simulink library "full_bridge_three_level_ttype_mosfet_based_model"  (R2026a)
settings: Solver=VariableStepAuto
undefined symbols (not defined in the file): tc
libraries: fl_lib x88, nesl_utility x56, ee_lib x8
(part 1 of 2)
settings Model: Creator=dbagn  LastModifiedBy=d.bagnara

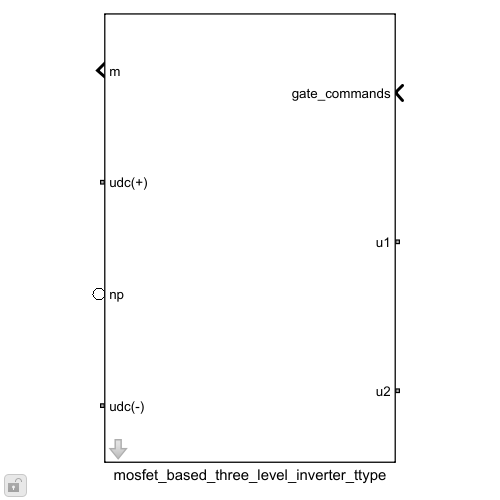
[thumbnail: Simulink's stored preview of the top-level diagram]
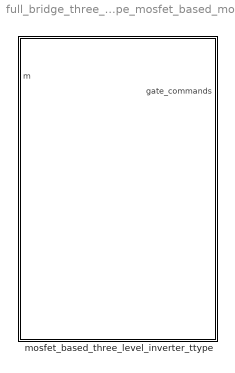
== system full_bridge_three_level_ttype_mosfet_based_model ==
  mosfet_based_three_level_inverter_ttype : Subsystem  mask{Vth_m=5.5, Rds_on_m=0.15e-3, Eon_m=200e-3, Eoff_m=300e-3, Erec_m=200e-3, Ion_sw_loss_m=900, Voff_sw_loss_m=900, Vdon_diode_m=2, Rdon_diode_m=0.15e-3, rth_mosfet_JH_m=0.018, rth_mosfet_HA_m=0.034, Csnubber_m=10e-9, Rsnubber_m=2200, JunctionTermalMass_m=2, mass_heatsink_m=0.15, specific_heat_m=880, Tambient_m=40, DThs_init_m=0, tc_m=tc}
      mask prompts: Vth_m "Vth (V)"; Rds_on_m "Rds_on (Ohm)"; Eon_m "Eon (J)"; Eoff_m "Eoff (J)"; Erec_m "Erec (J)"; Ion_sw_loss_m "Ion_sw_loss (A)"; Voff_sw_loss_m "Voff_sw_loss (V)"; Vdon_diode_m "Vdon_diode (V)"; Rdon_diode_m "Rdon_diode (Ohm)"; rth_mosfet_JH_m "rth_mosfet_JH (K/W)"; rth_mosfet_HA_m "rth_mosfet_HA  (K/W)"; Csnubber_m "Csnubber (F)"; Rsnubber_m "Rsnubber (Ohm)"; JunctionTermalMass_m "JunctionTermalMass (J/K)"; mass_heatsink_m "mass_heatsink (Kg)"; specific_heat_m "specific_heat (J/(K*Kg))"; Tambient_m "Tambient (Celsius)"; DThs_init_m "DThs_init (Celsius)"; tc_m "tc (s)"
      mask DialogControl inv Prompt: MOSFET
      mask DialogControl thermal Prompt: Thermal
      mask DialogControl sampling_time Prompt: Sampling time (s)

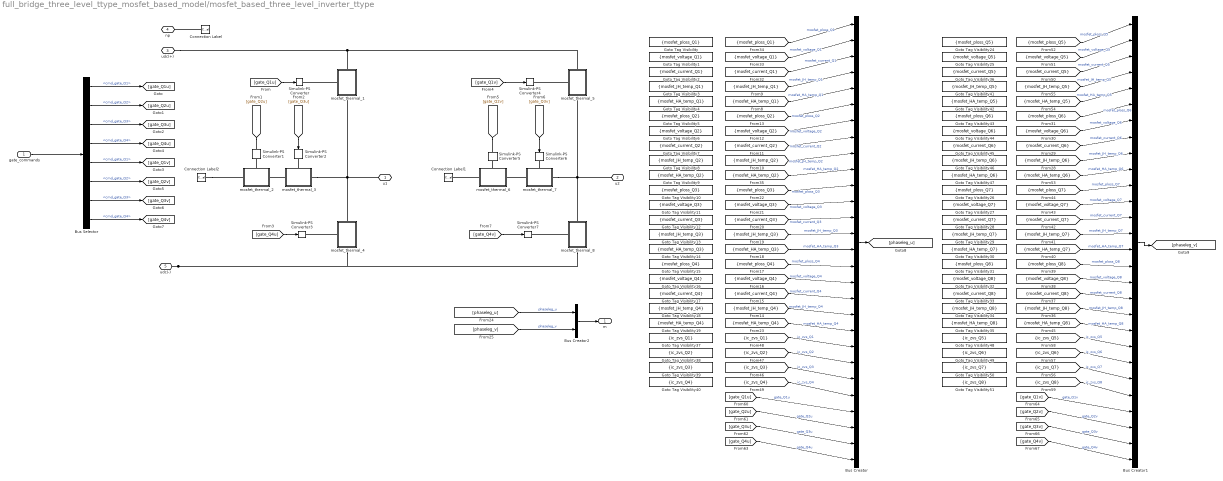
== system full_bridge_three_level_ttype_mosfet_based_model/mosfet_based_three_level_inverter_ttype ==
  gate_commands : Inport
  Bus Creator : BusCreator  Inputs=28
  Bus Creator1 : BusCreator  Inputs=28
  Bus Creator2 : BusCreator  Inputs=2
  Bus Selector : BusSelector  OutputSignals=gate_cmds_ph1.cmd_gate_Q1,gate_cmds_ph1.cmd_gate_Q2,gate_cmds_ph1.cmd_gate_Q3,gate_cmds_ph1.cmd_gate_Q4,gate_cmds_ph2.cmd_gate_Q1,gate_cmds_ph2.cmd_gate_Q2,gate_cmds_ph2.cmd_gate_Q3,gate_cmds_ph2.cmd_gate_Q4
  Connection Label : ConnectionLabel  Label=np
  Connection Label1 : ConnectionLabel  Label=np
  Connection Label2 : ConnectionLabel  Label=np
  Goto Tag Visibility : GotoTagVisibility  GotoTag=mosfet_ploss_Q1
  Goto Tag Visibility1 : GotoTagVisibility  GotoTag=mosfet_voltage_Q1
  Goto Tag Visibility10 : GotoTagVisibility  GotoTag=mosfet_ploss_Q3
  Goto Tag Visibility11 : GotoTagVisibility  GotoTag=mosfet_voltage_Q3
  Goto Tag Visibility12 : GotoTagVisibility  GotoTag=mosfet_current_Q3
  Goto Tag Visibility13 : GotoTagVisibility  GotoTag=mosfet_JH_temp_Q3
  Goto Tag Visibility14 : GotoTagVisibility  GotoTag=mosfet_HA_temp_Q3
  Goto Tag Visibility15 : GotoTagVisibility  GotoTag=mosfet_ploss_Q4
  Goto Tag Visibility16 : GotoTagVisibility  GotoTag=mosfet_voltage_Q4
  Goto Tag Visibility17 : GotoTagVisibility  GotoTag=mosfet_current_Q4
  Goto Tag Visibility18 : GotoTagVisibility  GotoTag=mosfet_JH_temp_Q4
  Goto Tag Visibility19 : GotoTagVisibility  GotoTag=mosfet_HA_temp_Q4
  Goto Tag Visibility2 : GotoTagVisibility  GotoTag=mosfet_current_Q1
  Goto Tag Visibility24 : GotoTagVisibility  GotoTag=mosfet_ploss_Q5
  Goto Tag Visibility25 : GotoTagVisibility  GotoTag=mosfet_voltage_Q5
  Goto Tag Visibility26 : GotoTagVisibility  GotoTag=mosfet_ploss_Q7
  Goto Tag Visibility27 : GotoTagVisibility  GotoTag=mosfet_voltage_Q7
  Goto Tag Visibility28 : GotoTagVisibility  GotoTag=mosfet_current_Q7
  Goto Tag Visibility29 : GotoTagVisibility  GotoTag=mosfet_JH_temp_Q7
  Goto Tag Visibility3 : GotoTagVisibility  GotoTag=mosfet_JH_temp_Q1
  Goto Tag Visibility30 : GotoTagVisibility  GotoTag=mosfet_HA_temp_Q7
  Goto Tag Visibility31 : GotoTagVisibility  GotoTag=mosfet_ploss_Q8
  Goto Tag Visibility32 : GotoTagVisibility  GotoTag=mosfet_voltage_Q8
  Goto Tag Visibility33 : GotoTagVisibility  GotoTag=mosfet_current_Q8
  Goto Tag Visibility34 : GotoTagVisibility  GotoTag=mosfet_JH_temp_Q8
  Goto Tag Visibility35 : GotoTagVisibility  GotoTag=mosfet_HA_temp_Q8
  Goto Tag Visibility36 : GotoTagVisibility  GotoTag=mosfet_current_Q5
  Goto Tag Visibility37 : GotoTagVisibility  GotoTag=ic_zvs_Q1
  Goto Tag Visibility38 : GotoTagVisibility  GotoTag=ic_zvs_Q2
  Goto Tag Visibility39 : GotoTagVisibility  GotoTag=ic_zvs_Q3
  Goto Tag Visibility4 : GotoTagVisibility  GotoTag=mosfet_HA_temp_Q1
  Goto Tag Visibility40 : GotoTagVisibility  GotoTag=ic_zvs_Q4
  Goto Tag Visibility41 : GotoTagVisibility  GotoTag=mosfet_JH_temp_Q5
  Goto Tag Visibility42 : GotoTagVisibility  GotoTag=mosfet_HA_temp_Q5
  Goto Tag Visibility43 : GotoTagVisibility  GotoTag=mosfet_ploss_Q6
  Goto Tag Visibility44 : GotoTagVisibility  GotoTag=mosfet_voltage_Q6
  Goto Tag Visibility45 : GotoTagVisibility  GotoTag=mosfet_current_Q6
  Goto Tag Visibility46 : GotoTagVisibility  GotoTag=mosfet_JH_temp_Q6
  Goto Tag Visibility47 : GotoTagVisibility  GotoTag=mosfet_HA_temp_Q6
  Goto Tag Visibility48 : GotoTagVisibility  GotoTag=ic_zvs_Q5
  Goto Tag Visibility49 : GotoTagVisibility  GotoTag=ic_zvs_Q6
  Goto Tag Visibility5 : GotoTagVisibility  GotoTag=mosfet_ploss_Q2
  Goto Tag Visibility50 : GotoTagVisibility  GotoTag=ic_zvs_Q7
  Goto Tag Visibility51 : GotoTagVisibility  GotoTag=ic_zvs_Q8
  Goto Tag Visibility6 : GotoTagVisibility  GotoTag=mosfet_voltage_Q2
  Goto Tag Visibility7 : GotoTagVisibility  GotoTag=mosfet_current_Q2
  Goto Tag Visibility8 : GotoTagVisibility  GotoTag=mosfet_JH_temp_Q2
  Goto Tag Visibility9 : GotoTagVisibility  GotoTag=mosfet_HA_temp_Q2
  Simulink-PS Converter{,1..7} (8 alike) : nesl_utility/Simulink-PS Converter  PhysicalDomain=network_engine_domain  SubClassName=ps_input  LeftPortType=input  RightPortType=output  PseudoPeriodic=off  Frequencies=[]  NoiseDistribution=none  NoiseParameters=[]  Unit=1  AffineConversion=on  FilteringAndDerivatives=provide  SimscapeFilterOrder=1  InputFilterTimeConstant=0.001  UdotUserProvided=0
  mosfet_thermal_1 : Subsystem
      settings: PortSchema="{\"entries\":[{\"content\":{\"sides\":[{\"content\":{\"connectorIds\":[\"LConn1\"]},\"type\":\"ConnectorPlacement.EquallySpacedRectSide\",\"uuid\":\"9277da8d-d460-43e6-8478-dd662f15d226\"},{\"content\":{\"connectorIds\":[],\"side\":\"RIGHT\"},\"type\":\"ConnectorPlacement.EquallySpacedRectSide\",\"uuid\":\"a7ece396-f1d9-4f4f-a05b-db1fc65d6e1d\"},{\"content\":{\"connectorIds\":[\"LConn2\"],\"side\":\"TOP\"},\"type\":\"ConnectorPlacement.EquallySpacedRectSide\",\"uuid\":\"fdd70777-e9cf-4317-afb6-cae87f75d5b0\"},{\"content\":{\"connectorIds\":[\"RConn1\"],\"side\":\"BOTTOM\"},\"type\":\"ConnectorPlacement.EquallySpacedRectSide\",\"uuid\":\"2353ed68-b1a1-4775-9ca9-31e268d5443b\"}]},\"type\":\"ConnectorPlacement.EquallySpacedConnector\",\"uuid\":\"d5479f4c-4e65-4791-adcb-73df11f88590\"}],\"packageUris\":[\"http://schema.mathworks.com/mf0/Connector/R2020b\"],\"version\":\"1.0\"}"
  mosfet_thermal_2 : Subsystem
      settings: PortSchema="{\"entries\":[{\"content\":{\"sides\":[{\"content\":{\"connectorIds\":[\"LConn1\"]},\"type\":\"ConnectorPlacement.EquallySpacedRectSide\",\"uuid\":\"9277da8d-d460-43e6-8478-dd662f15d226\"},{\"content\":{\"side\":\"RIGHT\"},\"type\":\"ConnectorPlacement.EquallySpacedRectSide\",\"uuid\":\"a7ece396-f1d9-4f4f-a05b-db1fc65d6e1d\"},{\"content\":{\"connectorIds\":[\"LConn2\"],\"side\":\"TOP\"},\"type\":\"ConnectorPlacement.EquallySpacedRectSide\",\"uuid\":\"fdd70777-e9cf-4317-afb6-cae87f75d5b0\"},{\"content\":{\"connectorIds\":[\"RConn1\"],\"side\":\"BOTTOM\"},\"type\":\"ConnectorPlacement.EquallySpacedRectSide\",\"uuid\":\"2353ed68-b1a1-4775-9ca9-31e268d5443b\"}]},\"type\":\"ConnectorPlacement.EquallySpacedConnector\",\"uuid\":\"d5479f4c-4e65-4791-adcb-73df11f88590\"}],\"packageUris\":[\"http://schema.mathworks.com/mf0/Connector/R2020b\"],\"version\":\"1.0\"}"
  mosfet_thermal_3 : Subsystem
      settings: PortSchema="{\"entries\":[{\"content\":{\"sides\":[{\"content\":{\"connectorIds\":[\"LConn1\"]},\"type\":\"ConnectorPlacement.EquallySpacedRectSide\",\"uuid\":\"9277da8d-d460-43e6-8478-dd662f15d226\"},{\"content\":{\"connectorIds\":[],\"side\":\"RIGHT\"},\"type\":\"ConnectorPlacement.EquallySpacedRectSide\",\"uuid\":\"a7ece396-f1d9-4f4f-a05b-db1fc65d6e1d\"},{\"content\":{\"connectorIds\":[\"LConn2\"],\"side\":\"TOP\"},\"type\":\"ConnectorPlacement.EquallySpacedRectSide\",\"uuid\":\"fdd70777-e9cf-4317-afb6-cae87f75d5b0\"},{\"content\":{\"connectorIds\":[\"RConn1\"],\"side\":\"BOTTOM\"},\"type\":\"ConnectorPlacement.EquallySpacedRectSide\",\"uuid\":\"2353ed68-b1a1-4775-9ca9-31e268d5443b\"}]},\"type\":\"ConnectorPlacement.EquallySpacedConnector\",\"uuid\":\"d5479f4c-4e65-4791-adcb-73df11f88590\"}],\"packageUris\":[\"http://schema.mathworks.com/mf0/Connector/R2020b\"],\"version\":\"1.0\"}"
  mosfet_thermal_4 : Subsystem
      settings: PortSchema="{\"entries\":[{\"content\":{\"sides\":[{\"content\":{\"connectorIds\":[\"LConn1\"]},\"type\":\"ConnectorPlacement.EquallySpacedRectSide\",\"uuid\":\"9277da8d-d460-43e6-8478-dd662f15d226\"},{\"content\":{\"connectorIds\":[],\"side\":\"RIGHT\"},\"type\":\"ConnectorPlacement.EquallySpacedRectSide\",\"uuid\":\"a7ece396-f1d9-4f4f-a05b-db1fc65d6e1d\"},{\"content\":{\"connectorIds\":[\"LConn2\"],\"side\":\"TOP\"},\"type\":\"ConnectorPlacement.EquallySpacedRectSide\",\"uuid\":\"fdd70777-e9cf-4317-afb6-cae87f75d5b0\"},{\"content\":{\"connectorIds\":[\"RConn1\"],\"side\":\"BOTTOM\"},\"type\":\"ConnectorPlacement.EquallySpacedRectSide\",\"uuid\":\"2353ed68-b1a1-4775-9ca9-31e268d5443b\"}]},\"type\":\"ConnectorPlacement.EquallySpacedConnector\",\"uuid\":\"d5479f4c-4e65-4791-adcb-73df11f88590\"}],\"packageUris\":[\"http://schema.mathworks.com/mf0/Connector/R2020b\"],\"version\":\"1.0\"}"
  mosfet_thermal_5 : Subsystem
      settings: PortSchema="{\"entries\":[{\"content\":{\"sides\":[{\"content\":{\"connectorIds\":[\"LConn1\"]},\"type\":\"ConnectorPlacement.EquallySpacedRectSide\",\"uuid\":\"9277da8d-d460-43e6-8478-dd662f15d226\"},{\"content\":{\"connectorIds\":[],\"side\":\"RIGHT\"},\"type\":\"ConnectorPlacement.EquallySpacedRectSide\",\"uuid\":\"a7ece396-f1d9-4f4f-a05b-db1fc65d6e1d\"},{\"content\":{\"connectorIds\":[\"LConn2\"],\"side\":\"TOP\"},\"type\":\"ConnectorPlacement.EquallySpacedRectSide\",\"uuid\":\"fdd70777-e9cf-4317-afb6-cae87f75d5b0\"},{\"content\":{\"connectorIds\":[\"RConn1\"],\"side\":\"BOTTOM\"},\"type\":\"ConnectorPlacement.EquallySpacedRectSide\",\"uuid\":\"2353ed68-b1a1-4775-9ca9-31e268d5443b\"}]},\"type\":\"ConnectorPlacement.EquallySpacedConnector\",\"uuid\":\"d5479f4c-4e65-4791-adcb-73df11f88590\"}],\"packageUris\":[\"http://schema.mathworks.com/mf0/Connector/R2020b\"],\"version\":\"1.0\"}"
  mosfet_thermal_6 : Subsystem
      settings: PortSchema="{\"entries\":[{\"content\":{\"sides\":[{\"content\":{\"connectorIds\":[\"LConn1\"]},\"type\":\"ConnectorPlacement.EquallySpacedRectSide\",\"uuid\":\"9277da8d-d460-43e6-8478-dd662f15d226\"},{\"content\":{\"connectorIds\":[],\"side\":\"RIGHT\"},\"type\":\"ConnectorPlacement.EquallySpacedRectSide\",\"uuid\":\"a7ece396-f1d9-4f4f-a05b-db1fc65d6e1d\"},{\"content\":{\"connectorIds\":[\"LConn2\"],\"side\":\"TOP\"},\"type\":\"ConnectorPlacement.EquallySpacedRectSide\",\"uuid\":\"fdd70777-e9cf-4317-afb6-cae87f75d5b0\"},{\"content\":{\"connectorIds\":[\"RConn1\"],\"side\":\"BOTTOM\"},\"type\":\"ConnectorPlacement.EquallySpacedRectSide\",\"uuid\":\"2353ed68-b1a1-4775-9ca9-31e268d5443b\"}]},\"type\":\"ConnectorPlacement.EquallySpacedConnector\",\"uuid\":\"d5479f4c-4e65-4791-adcb-73df11f88590\"}],\"packageUris\":[\"http://schema.mathworks.com/mf0/Connector/R2020b\"],\"version\":\"1.0\"}"
  mosfet_thermal_7 : Subsystem
      settings: PortSchema="{\"entries\":[{\"content\":{\"sides\":[{\"content\":{\"connectorIds\":[\"LConn1\"]},\"type\":\"ConnectorPlacement.EquallySpacedRectSide\",\"uuid\":\"9277da8d-d460-43e6-8478-dd662f15d226\"},{\"content\":{\"connectorIds\":[],\"side\":\"RIGHT\"},\"type\":\"ConnectorPlacement.EquallySpacedRectSide\",\"uuid\":\"a7ece396-f1d9-4f4f-a05b-db1fc65d6e1d\"},{\"content\":{\"connectorIds\":[\"LConn2\"],\"side\":\"TOP\"},\"type\":\"ConnectorPlacement.EquallySpacedRectSide\",\"uuid\":\"fdd70777-e9cf-4317-afb6-cae87f75d5b0\"},{\"content\":{\"connectorIds\":[\"RConn1\"],\"side\":\"BOTTOM\"},\"type\":\"ConnectorPlacement.EquallySpacedRectSide\",\"uuid\":\"2353ed68-b1a1-4775-9ca9-31e268d5443b\"}]},\"type\":\"ConnectorPlacement.EquallySpacedConnector\",\"uuid\":\"d5479f4c-4e65-4791-adcb-73df11f88590\"}],\"packageUris\":[\"http://schema.mathworks.com/mf0/Connector/R2020b\"],\"version\":\"1.0\"}"
  mosfet_thermal_8 : Subsystem
      settings: PortSchema="{\"entries\":[{\"content\":{\"sides\":[{\"content\":{\"connectorIds\":[\"LConn1\"]},\"type\":\"ConnectorPlacement.EquallySpacedRectSide\",\"uuid\":\"9277da8d-d460-43e6-8478-dd662f15d226\"},{\"content\":{\"connectorIds\":[],\"side\":\"RIGHT\"},\"type\":\"ConnectorPlacement.EquallySpacedRectSide\",\"uuid\":\"a7ece396-f1d9-4f4f-a05b-db1fc65d6e1d\"},{\"content\":{\"connectorIds\":[\"LConn2\"],\"side\":\"TOP\"},\"type\":\"ConnectorPlacement.EquallySpacedRectSide\",\"uuid\":\"fdd70777-e9cf-4317-afb6-cae87f75d5b0\"},{\"content\":{\"connectorIds\":[\"RConn1\"],\"side\":\"BOTTOM\"},\"type\":\"ConnectorPlacement.EquallySpacedRectSide\",\"uuid\":\"2353ed68-b1a1-4775-9ca9-31e268d5443b\"}]},\"type\":\"ConnectorPlacement.EquallySpacedConnector\",\"uuid\":\"d5479f4c-4e65-4791-adcb-73df11f88590\"}],\"packageUris\":[\"http://schema.mathworks.com/mf0/Connector/R2020b\"],\"version\":\"1.0\"}"
  u1 : PMIOPort  Side=Left
  u2 : PMIOPort  Port=2  Side=Left
  udc(+) : PMIOPort  Port=3  Side=Right
  np : PMIOPort  Port=4  Side=Right
  udc(-) : PMIOPort  Port=5  Side=Right
  m : Outport
  wires:
  [gate_Q4u] -> Simulink-PS Converter3/1
  [gate_Q3u] -> Simulink-PS Converter2/1
  [gate_Q2u] -> Simulink-PS Converter1/1
  [gate_Q1u] -> Simulink-PS Converter/1
  [gate_Q1v] -> Simulink-PS Converter4/1
  [gate_Q2v] -> Simulink-PS Converter5/1
  [gate_Q3v] -> Simulink-PS Converter6/1
  [gate_Q4v] -> Simulink-PS Converter7/1
  gate_commands/1 -> Bus Selector/1
  Bus Selector/1 -> [gate_Q1u]  "<cmd_gate_Q1>"
  Bus Selector/2 -> [gate_Q2u]  "<cmd_gate_Q2>"
  Bus Selector/3 -> [gate_Q3u]  "<cmd_gate_Q3>"
  Bus Selector/4 -> [gate_Q4u]  "<cmd_gate_Q4>"
  Bus Selector/5 -> [gate_Q1v]  "<cmd_gate_Q1>"
  Bus Selector/6 -> [gate_Q2v]  "<cmd_gate_Q2>"
  Bus Selector/7 -> [gate_Q3v]  "<cmd_gate_Q3>"
  Bus Selector/8 -> [gate_Q4v]  "<cmd_gate_Q4>"
  [mosfet_ploss_Q1] -> Bus Creator/1  "mosfet_ploss_Q1"
  [mosfet_voltage_Q1] -> Bus Creator/2  "mosfet_voltage_Q1"
  [mosfet_current_Q1] -> Bus Creator/3  "mosfet_current_Q1"
  [mosfet_JH_temp_Q1] -> Bus Creator/4  "mosfet_JH_temp_Q1"
  [mosfet_HA_temp_Q1] -> Bus Creator/5  "mosfet_HA_temp_Q1"
  [mosfet_ploss_Q2] -> Bus Creator/6  "mosfet_ploss_Q2"
  [mosfet_voltage_Q2] -> Bus Creator/7  "mosfet_voltage_Q2"
  [mosfet_current_Q2] -> Bus Creator/8  "mosfet_current_Q2"
  [mosfet_JH_temp_Q2] -> Bus Creator/9  "mosfet_JH_temp_Q2"
  [mosfet_HA_temp_Q2] -> Bus Creator/10  "mosfet_HA_temp_Q2"
  [ic_zvs_Q4] -> Bus Creator/24  "ic_zvs_Q4"
  [gate_Q1u] -> Bus Creator/25  "gate_Q1u"
  [gate_Q2u] -> Bus Creator/26  "gate_Q2u"
  [gate_Q3u] -> Bus Creator/27  "gate_Q3u"
  [gate_Q4u] -> Bus Creator/28  "gate_Q4u"
  [ic_zvs_Q3] -> Bus Creator/23  "ic_zvs_Q3"
  [ic_zvs_Q2] -> Bus Creator/22  "ic_zvs_Q2"
  [ic_zvs_Q1] -> Bus Creator/21  "ic_zvs_Q1"
  [mosfet_HA_temp_Q4] -> Bus Creator/20  "mosfet_HA_temp_Q4"
  [mosfet_JH_temp_Q4] -> Bus Creator/19  "mosfet_JH_temp_Q4"
  [mosfet_current_Q4] -> Bus Creator/18  "mosfet_current_Q4"
  [mosfet_voltage_Q4] -> Bus Creator/17  "mosfet_voltage_Q4"
  [mosfet_ploss_Q4] -> Bus Creator/16  "mosfet_ploss_Q4"
  [mosfet_HA_temp_Q3] -> Bus Creator/15  "mosfet_HA_temp_Q3"
  [mosfet_JH_temp_Q3] -> Bus Creator/14  "mosfet_JH_temp_Q3"
  [mosfet_current_Q3] -> Bus Creator/13  "mosfet_current_Q3"
  [mosfet_voltage_Q3] -> Bus Creator/12  "mosfet_voltage_Q3"
  [mosfet_ploss_Q3] -> Bus Creator/11  "mosfet_ploss_Q3"
  [mosfet_voltage_Q5] -> Bus Creator1/2  "mosfet_voltage_Q5"
  [mosfet_ploss_Q5] -> Bus Creator1/1  "mosfet_ploss_Q5"
  [mosfet_current_Q5] -> Bus Creator1/3  "mosfet_current_Q5"
  [mosfet_JH_temp_Q5] -> Bus Creator1/4  "mosfet_JH_temp_Q5"
  [mosfet_HA_temp_Q5] -> Bus Creator1/5  "mosfet_HA_temp_Q5"
  [mosfet_ploss_Q6] -> Bus Creator1/6  "mosfet_ploss_Q6"
  [mosfet_voltage_Q6] -> Bus Creator1/7  "mosfet_voltage_Q6"
  [mosfet_current_Q6] -> Bus Creator1/8  "mosfet_current_Q6"
  [mosfet_JH_temp_Q6] -> Bus Creator1/9  "mosfet_JH_temp_Q6"
  [mosfet_HA_temp_Q6] -> Bus Creator1/10  "mosfet_HA_temp_Q6"
  [mosfet_ploss_Q7] -> Bus Creator1/11  "mosfet_ploss_Q7"
  [mosfet_voltage_Q7] -> Bus Creator1/12  "mosfet_voltage_Q7"
  [mosfet_current_Q7] -> Bus Creator1/13  "mosfet_current_Q7"
  [mosfet_JH_temp_Q7] -> Bus Creator1/14  "mosfet_JH_temp_Q7"
  [mosfet_HA_temp_Q7] -> Bus Creator1/15  "mosfet_HA_temp_Q7"
  [mosfet_ploss_Q8] -> Bus Creator1/16  "mosfet_ploss_Q8"
  [mosfet_voltage_Q8] -> Bus Creator1/17  "mosfet_voltage_Q8"
  [mosfet_current_Q8] -> Bus Creator1/18  "mosfet_current_Q8"
  [mosfet_JH_temp_Q8] -> Bus Creator1/19  "mosfet_JH_temp_Q8"
  [mosfet_HA_temp_Q8] -> Bus Creator1/20  "mosfet_HA_temp_Q8"
  [ic_zvs_Q5] -> Bus Creator1/21  "ic_zvs_Q5"
  [ic_zvs_Q6] -> Bus Creator1/22  "ic_zvs_Q6"
  [ic_zvs_Q7] -> Bus Creator1/23  "ic_zvs_Q7"
  [ic_zvs_Q8] -> Bus Creator1/24  "ic_zvs_Q8"
  [gate_Q1v] -> Bus Creator1/25  "gate_Q1v"
  [gate_Q2v] -> Bus Creator1/26  "gate_Q2v"
  [gate_Q3v] -> Bus Creator1/27  "gate_Q3v"
  [gate_Q4v] -> Bus Creator1/28  "gate_Q4v"
  Bus Creator/1 -> [phaseleg_u]
  [phaseleg_u] -> Bus Creator2/1  "phaseleg_u"
  Bus Creator1/1 -> [phaseleg_v]
  [phaseleg_v] -> Bus Creator2/2  "phaseleg_v"
  Bus Creator2/1 -> m/1
  connections:
  udc(+)/RConn1 -- mosfet_thermal_5/LConn2 -- mosfet_thermal_1/LConn2
  mosfet_thermal_4/LConn1 -- Simulink-PS Converter3/RConn1
  mosfet_thermal_3/LConn1 -- Simulink-PS Converter2/RConn1
  mosfet_thermal_2/LConn1 -- Simulink-PS Converter1/RConn1
  mosfet_thermal_1/LConn1 -- Simulink-PS Converter/RConn1
  mosfet_thermal_6/LConn1 -- Simulink-PS Converter5/RConn1
  mosfet_thermal_5/LConn1 -- Simulink-PS Converter4/RConn1
  mosfet_thermal_7/LConn1 -- Simulink-PS Converter6/RConn1
  mosfet_thermal_8/LConn1 -- Simulink-PS Converter7/RConn1
  udc(-)/RConn1 -- mosfet_thermal_8/RConn1 -- mosfet_thermal_4/RConn1
  Connection Label/LConn1 -- np/RConn1
  mosfet_thermal_3/RConn1 -- mosfet_thermal_2/RConn1
  Connection Label2/LConn1 -- mosfet_thermal_2/LConn2
  mosfet_thermal_3/LConn2 -- mosfet_thermal_4/LConn2 -- mosfet_thermal_1/RConn1 -- u1/RConn1
  mosfet_thermal_6/LConn2 -- Connection Label1/LConn1
  mosfet_thermal_7/RConn1 -- mosfet_thermal_6/RConn1
  mosfet_thermal_7/LConn2 -- u2/RConn1 -- mosfet_thermal_8/LConn2 -- mosfet_thermal_5/RConn1

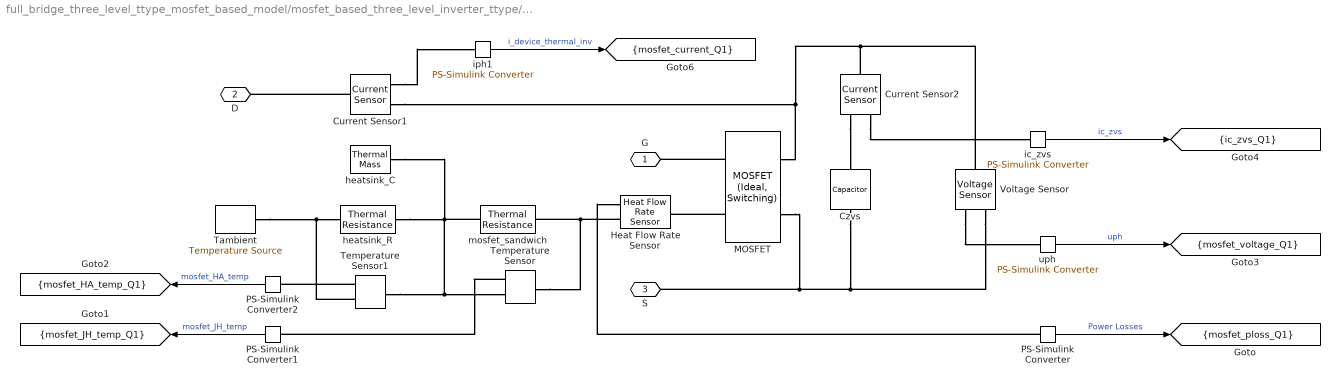
== system full_bridge_three_level_ttype_mosfet_based_model/mosfet_based_three_level_inverter_ttype/mosfet_thermal_1 ==
  Current Sensor1 : fl_lib/Electrical/Electrical Sensors/Current Sensor
  Current Sensor2 : fl_lib/Electrical/Electrical Sensors/Current Sensor
  Czvs : fl_lib/Electrical/Electrical Elements/Capacitor  c=Csnubber_m F  r=Rsnubber_m Ohm  g=0 1/Ohm  i_specify=off  i_priority=None  i=0 A  i_nominal_specify=off  i_nominal_value=1  i_nominal_unit=A  v_specify=off  v_priority=None  v=0 V  v_nominal_specify=off  v_nominal_value=1  v_nominal_unit=V  vc_specify=off  vc_priority=High  vc=0 V  vc_nominal_specify=off  vc_nominal_value=1  vc_nominal_unit=V
  Heat Flow Rate Sensor : fl_lib/Thermal/Thermal Sensors/Heat Flow Rate Sensor
  MOSFET : ee_lib/Semiconductors & Converters/MOSFET (Ideal, Switching)  port_option=ee.enum.controlport.ps  Rds=Rds_on_m Ohm  Goff=1e-6 1/Ohm  Vth=Vth_m V  diode_param=ee.enum.converters.protectiondiode.nodynamics  diode_Vf=Vdon_diode_m V  diode_Ron=Rdon_diode_m Ohm  diode_Goff=1e-5 1/Ohm  diode_C=50e-9 F  diode_iRM=-235 A  diode_iF=300 A  diode_idot=-50 A/us  diode_trr_param=ee.enum.converters.diodeReverseParam.trr_factor  diode_trr_factor=3  diode_trr=15 us  diode_Qrr=1500 s*uA  ids_specify=off  ids_priority=None  ids=0 A  ids_nominal_specify=off  ids_nominal_value=1  ids_nominal_unit=A  vds_specify=off  vds_priority=None  vds=0 V  vds_nominal_specify=off  vds_nominal_value=1  vds_nominal_unit=V  vgs_specify=off  vgs_priority=None  vgs=0 V  vgs_nominal_specify=off  vgs_nominal_value=1  vgs_nominal_unit=V  thermal_loss_option=ee.enum.converters.thermalLossOption.constantvalues  Von_data=[0, 1.8, 3.2, 6, 10, 16; 0, 2, 5.5, 9.5, 15, 25] V  Tj=[298.15, 448.15] K  Iout_data=[0, 20, 40, 60, 80, 100] A  tabulateWithVds=false  Eon_data=[0, 55.04, 124.57, 235.53, 362.12; 0, 71.25, 161.25, 304.88, 468.75] * 1e-6 J  Eoff_data=[0, 18, 30, 56.1, 76.5; 0, 22.5, 37.5, 70.13, 95.63] * 1e-6 J  Eon_data_3D=[zeros(2, 5, 3)] J  Eoff_data_3D=[zeros(2, 5, 3)] J  Tj_loss=[298.15, 448.15] K  Iout_data_loss=[0, 10, 20, 30, 40] A  Vds_loss=[0, 150, 300] V  Eon_scalar=Eon_m J  Eoff_scalar=Eoff_m J  Voff=Voff_sw_loss_m V  Iout_scalar=Ion_sw_loss_m A  useCurrentFromPreviousCycle=true  useVoltageFromPreviousCycle=true  diodeModelType=ee.enum.converters.diodeModelType.pwl  diodeTableType=ee.enum.diode.tableType.IfMat  diode_ReverseIVType=ee.enum.diode.diodeReverseIV.constant  diode_IfMat=[.07, .12, .19, 1.75, 4.24, 7.32, 11.2; .16, .3, .72, 2.14, 4.02, 6.35, 9.12] A  diode_VfMat=[.9, 1.15, 1.25, 1.5, 1.75, 2.17, 2.6, 2.85; .58, .68, .75, 1.1, 1.38, 1.77, 2.27, 2.7] V  diode_TjVec=[25, 125] degC  diode_VfVec=[.5, .7, .9, 1.3, 1.7, 2.1, 2.5] V  diode_IfVec=[.1, .2, .5, 1, 2, 4, 7, 10] A  diode_IrMat=[1e-06, 2e-06, 5e-06, 1e-05, 2.5e-05, 5e-05, .0001; 2e-06, 5e-06, 1e-05, 4e-05, 8e-05, .0002, .0005] A  diode_VrMat=[10, 100, 200, 250, 300, 325, 350; 10, 70, 160, 220, 270, 300, 320] V  diode_VrVec=[10, 20, 40, 50, 70, 80, 100] V  diode_IrVec=[1e-06, 2e-06, 5e-06, 1e-05, 2e-05, 5e-05, .0001] A  diode_Vr=-600 V  diode_Ls=150 nH  diode_Erec=0.03 J  diode_rec_loss_model=ee.enum.diode.reverseRecoveryModel.fixed  diode_ErecVal=0 J  diode_scaleWithIandV=false  diode_ErecMat=zeros(2, 3) J  diodeErecMat3D=zeros(2, 3, 2) J  diode_TjrecVec=[298.15, 398.15] K  diode_IfrecVec=[.1, 1, 10] A  diodeVrecVec=[0, 100] V  diode_IrecVal=10 A  diode_VrecVal=10 V  diode_tFilter=1 / 1000 / 100 s  separateThermalPortForDiode=false  thermal_network_parameterization=ee.enum.thermalNetworkTopology.external  Rth=[.03, .2] K/W  Rth_Cauer=[.03, .1, .2] K/W  Rth_Foster=[.03, .2] K/W  thermal_mass_parameterization=ee.enum.thermalNetwork.thermalmass  thermal_mass=[3, 25] J/K  thermal_mass_Cauer=[3, 10, 25] J/K  thermal_mass_Foster=[33, 50] J/K  thermal_time_constant=[.1, 5] s  thermal_time_constant_Cauer=[.1, 1, 5] s  thermal_time_constant_Foster=[1, 10] s  thermal_mass_initial_temperatures=[80, 80] degC  thermal_mass_initial_temperatures_Cauer=[25, 25, 25] degC  junction_thermal_mass=JunctionTermalMass_m J/K  Tvec_initial_Foster=[25, 25, 25, 25] degC  RthDiode=[.03, .2] K/W  RthCauerDiode=[.03, .1, .2] K/W  RthFosterDiode=[.03, .2] K/W  thermalMassDiode=[3, 25] J/K  thermalMassCauerDiode=[3, 10, 25] J/K  thermalMassFosterDiode=[33, 50] J/K  thermalTauDiode=[.1, 5] s  thermalTauCauerDiode=[.1, 1, 5] s  thermalTauFosterDiode=[1, 10] s  thermalMassInitTempDiode=[25, 25] degC  thermalMassInitTempCauerDiode=[25, 25, 25] degC  junctionthermalMassDiode=0.1 J/K  TVecInitialFosterDiode=[25, 25, 25, 25] degC  no_thermal_network=0  mosfet_junction_temperature_specify=on  mosfet_junction_temperature_priority=High  mosfet_junction_temperature=Tambient_m+DThs_init_m degC  mosfet_junction_temperature_nominal_specify=off  mosfet_junction_temperature_nominal_value=1  mosfet_junction_temperature_nominal_unit=degC  diode_junction_temperature_specify=off  diode_junction_temperature_priority=None  diode_junction_temperature=25 degC  diode_junction_temperature_nominal_specify=off  diode_junction_temperature_nominal_value=1  diode_junction_temperature_nominal_unit=degC  Qj_specify=off  Qj_priority=None  Qj=0 W  Qj_nominal_specify=off  Qj_nominal_value=1  Qj_nominal_unit=W  accumulatedSwitchingLosses_specify=off  accumulatedSwitchingLosses_priority=None  accumulatedSwitchingLosses=0 J
  PS-Simulink Converter : nesl_utility/PS-Simulink Converter  PhysicalDomain=network_engine_domain  SubClassName=ps_output  LeftPortType=input  RightPortType=output  PseudoPeriodic=off  Frequencies=[]  VectorFormat=1-D array  Unit=W  AffineConversion=off
  PS-Simulink Converter1 : nesl_utility/PS-Simulink Converter  PhysicalDomain=network_engine_domain  SubClassName=ps_output  LeftPortType=input  RightPortType=output  PseudoPeriodic=off  Frequencies=[]  VectorFormat=1-D array  Unit=degC  AffineConversion=off
  PS-Simulink Converter2 : nesl_utility/PS-Simulink Converter  PhysicalDomain=network_engine_domain  SubClassName=ps_output  LeftPortType=input  RightPortType=output  PseudoPeriodic=off  Frequencies=[]  VectorFormat=1-D array  Unit=degC  AffineConversion=off
  Tambient : fl_lib/Thermal/Thermal Sources/Temperature Source  temperature=Tambient_m degC
  Temperature Sensor : fl_lib/Thermal/Thermal Sensors/Temperature Sensor  temperature_measure=foundation.enum.MeasurementReference.difference
  Temperature Sensor1 : fl_lib/Thermal/Thermal Sensors/Temperature Sensor  temperature_measure=foundation.enum.MeasurementReference.difference
  Voltage Sensor : fl_lib/Electrical/Electrical Sensors/Voltage Sensor
  heatsink_C : fl_lib/Thermal/Thermal Elements/Thermal Mass  mass_type=foundation.enum.constant_variable.constant  mass=mass_heatsink_m kg  sp_heat=specific_heat_m J/(K*kg)  mass_min=1e-6 kg  num_ports=foundation.enum.numPorts2.one  m_specify=off  m_priority=High  m=1 kg  m_nominal_specify=off  m_nominal_value=1  m_nominal_unit=kg  T_specify=on  T_priority=High  T=DThs_init_m+Tambient_m degC  T_nominal_specify=off  T_nominal_value=1  T_nominal_unit=K  Q_specify=off  Q_priority=High  Q=0 W  Q_nominal_specify=off  Q_nominal_value=1  Q_nominal_unit=W
  heatsink_R : fl_lib/Thermal/Thermal Elements/Thermal Resistance  resistance=rth_mosfet_HA_m K/W  T_specify=off  T_priority=High  T=0 deltadegC  T_nominal_specify=off  T_nominal_value=1  T_nominal_unit=K  Q_specify=off  Q_priority=None  Q=0 W  Q_nominal_specify=off  Q_nominal_value=1  Q_nominal_unit=W
  ic_zvs : nesl_utility/PS-Simulink Converter  PhysicalDomain=network_engine_domain  SubClassName=ps_output  LeftPortType=input  RightPortType=output  PseudoPeriodic=off  Frequencies=[]  VectorFormat=1-D array  Unit=A  AffineConversion=off
  iph1 : nesl_utility/PS-Simulink Converter  PhysicalDomain=network_engine_domain  SubClassName=ps_output  LeftPortType=input  RightPortType=output  PseudoPeriodic=off  Frequencies=[]  VectorFormat=1-D array  Unit=A  AffineConversion=off
  mosfet_sandwich : fl_lib/Thermal/Thermal Elements/Thermal Resistance  resistance=rth_mosfet_JH_m K/W  T_specify=off  T_priority=High  T=0 degC  T_nominal_specify=off  T_nominal_value=1  T_nominal_unit=K  Q_specify=off  Q_priority=None  Q=0 W  Q_nominal_specify=off  Q_nominal_value=1  Q_nominal_unit=W
  uph : nesl_utility/PS-Simulink Converter  PhysicalDomain=network_engine_domain  SubClassName=ps_output  LeftPortType=input  RightPortType=output  PseudoPeriodic=off  Frequencies=[]  VectorFormat=1-D array  Unit=V  AffineConversion=off
  G : PMIOPort  Side=Left
  D : PMIOPort  Port=2  Side=Left
  S : PMIOPort  Port=3  Side=Right
  tag scope: ic_zvs_Q1=scoped, mosfet_HA_temp_Q1=scoped, mosfet_JH_temp_Q1=scoped, mosfet_current_Q1=scoped, mosfet_ploss_Q1=scoped, mosfet_voltage_Q1=scoped
  wires:
  PS-Simulink Converter/1 -> [mosfet_ploss_Q1]  "Power Losses"
  PS-Simulink Converter2/1 -> [mosfet_HA_temp_Q1]  "mosfet_HA_temp"
  PS-Simulink Converter1/1 -> [mosfet_JH_temp_Q1]  "mosfet_JH_temp"
  iph1/1 -> [mosfet_current_Q1]  "i_device_thermal_inv"
  uph/1 -> [mosfet_voltage_Q1]  "uph"
  ic_zvs/1 -> [ic_zvs_Q1]  "ic_zvs"
  connections:
  S/RConn1 -- Czvs/RConn1 -- Voltage Sensor/RConn2 -- MOSFET/RConn2
  MOSFET/LConn1 -- G/RConn1
  PS-Simulink Converter/LConn1 -- Heat Flow Rate Sensor/RConn1
  Temperature Sensor/LConn1 -- Heat Flow Rate Sensor/RConn2 -- mosfet_sandwich/LConn1
  mosfet_sandwich/RConn1 -- heatsink_C/LConn1 -- heatsink_R/LConn1 -- Temperature Sensor1/LConn1 -- Temperature Sensor/RConn1
  Temperature Sensor/RConn2 -- PS-Simulink Converter1/LConn1
  Tambient/LConn1 -- Temperature Sensor1/RConn1 -- heatsink_R/RConn1
  Temperature Sensor1/RConn2 -- PS-Simulink Converter2/LConn1
  MOSFET/LConn2 -- Heat Flow Rate Sensor/LConn1
  Current Sensor1/LConn1 -- D/RConn1
  Current Sensor1/RConn2 -- Current Sensor2/LConn1 -- Voltage Sensor/LConn1 -- MOSFET/RConn1
  Current Sensor1/RConn1 -- iph1/LConn1
  Voltage Sensor/RConn1 -- uph/LConn1
  Current Sensor2/RConn2 -- Czvs/LConn1
  Current Sensor2/RConn1 -- ic_zvs/LConn1

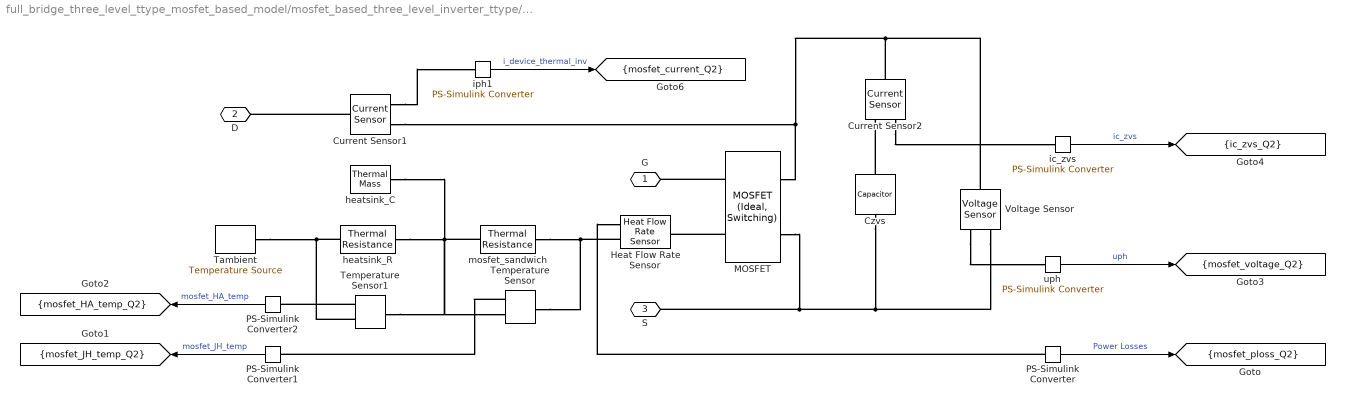
== system full_bridge_three_level_ttype_mosfet_based_model/mosfet_based_three_level_inverter_ttype/mosfet_thermal_2 ==
  Current Sensor1 : fl_lib/Electrical/Electrical Sensors/Current Sensor
  Current Sensor2 : fl_lib/Electrical/Electrical Sensors/Current Sensor
  Czvs : fl_lib/Electrical/Electrical Elements/Capacitor  c=Csnubber_m F  r=Rsnubber_m Ohm  g=0 1/Ohm  i_specify=off  i_priority=None  i=0 A  i_nominal_specify=off  i_nominal_value=1  i_nominal_unit=A  v_specify=off  v_priority=None  v=0 V  v_nominal_specify=off  v_nominal_value=1  v_nominal_unit=V  vc_specify=off  vc_priority=High  vc=0 V  vc_nominal_specify=off  vc_nominal_value=1  vc_nominal_unit=V
  Heat Flow Rate Sensor : fl_lib/Thermal/Thermal Sensors/Heat Flow Rate Sensor
  MOSFET : ee_lib/Semiconductors & Converters/MOSFET (Ideal, Switching)  port_option=ee.enum.controlport.ps  Rds=Rds_on_m Ohm  Goff=1e-6 1/Ohm  Vth=Vth_m V  diode_param=ee.enum.converters.protectiondiode.nodynamics  diode_Vf=Vdon_diode_m V  diode_Ron=Rdon_diode_m Ohm  diode_Goff=1e-5 1/Ohm  diode_C=50e-9 F  diode_iRM=-235 A  diode_iF=300 A  diode_idot=-50 A/us  diode_trr_param=ee.enum.converters.diodeReverseParam.trr_factor  diode_trr_factor=3  diode_trr=15 us  diode_Qrr=1500 s*uA  ids_specify=off  ids_priority=None  ids=0 A  ids_nominal_specify=off  ids_nominal_value=1  ids_nominal_unit=A  vds_specify=off  vds_priority=None  vds=0 V  vds_nominal_specify=off  vds_nominal_value=1  vds_nominal_unit=V  vgs_specify=off  vgs_priority=None  vgs=0 V  vgs_nominal_specify=off  vgs_nominal_value=1  vgs_nominal_unit=V  thermal_loss_option=ee.enum.converters.thermalLossOption.constantvalues  Von_data=[0, 1.8, 3.2, 6, 10, 16; 0, 2, 5.5, 9.5, 15, 25] V  Tj=[298.15, 448.15] K  Iout_data=[0, 20, 40, 60, 80, 100] A  tabulateWithVds=false  Eon_data=[0, 55.04, 124.57, 235.53, 362.12; 0, 71.25, 161.25, 304.88, 468.75] * 1e-6 J  Eoff_data=[0, 18, 30, 56.1, 76.5; 0, 22.5, 37.5, 70.13, 95.63] * 1e-6 J  Eon_data_3D=[zeros(2, 5, 3)] J  Eoff_data_3D=[zeros(2, 5, 3)] J  Tj_loss=[298.15, 448.15] K  Iout_data_loss=[0, 10, 20, 30, 40] A  Vds_loss=[0, 150, 300] V  Eon_scalar=Eon_m J  Eoff_scalar=Eoff_m J  Voff=Voff_sw_loss_m V  Iout_scalar=Ion_sw_loss_m A  useCurrentFromPreviousCycle=true  useVoltageFromPreviousCycle=true  diodeModelType=ee.enum.converters.diodeModelType.pwl  diodeTableType=ee.enum.diode.tableType.IfMat  diode_ReverseIVType=ee.enum.diode.diodeReverseIV.constant  diode_IfMat=[.07, .12, .19, 1.75, 4.24, 7.32, 11.2; .16, .3, .72, 2.14, 4.02, 6.35, 9.12] A  diode_VfMat=[.9, 1.15, 1.25, 1.5, 1.75, 2.17, 2.6, 2.85; .58, .68, .75, 1.1, 1.38, 1.77, 2.27, 2.7] V  diode_TjVec=[25, 125] degC  diode_VfVec=[.5, .7, .9, 1.3, 1.7, 2.1, 2.5] V  diode_IfVec=[.1, .2, .5, 1, 2, 4, 7, 10] A  diode_IrMat=[1e-06, 2e-06, 5e-06, 1e-05, 2.5e-05, 5e-05, .0001; 2e-06, 5e-06, 1e-05, 4e-05, 8e-05, .0002, .0005] A  diode_VrMat=[10, 100, 200, 250, 300, 325, 350; 10, 70, 160, 220, 270, 300, 320] V  diode_VrVec=[10, 20, 40, 50, 70, 80, 100] V  diode_IrVec=[1e-06, 2e-06, 5e-06, 1e-05, 2e-05, 5e-05, .0001] A  diode_Vr=-600 V  diode_Ls=150 nH  diode_Erec=0.03 J  diode_rec_loss_model=ee.enum.diode.reverseRecoveryModel.fixed  diode_ErecVal=0 J  diode_scaleWithIandV=false  diode_ErecMat=zeros(2, 3) J  diodeErecMat3D=zeros(2, 3, 2) J  diode_TjrecVec=[298.15, 398.15] K  diode_IfrecVec=[.1, 1, 10] A  diodeVrecVec=[0, 100] V  diode_IrecVal=10 A  diode_VrecVal=10 V  diode_tFilter=1 / 1000 / 100 s  separateThermalPortForDiode=false  thermal_network_parameterization=ee.enum.thermalNetworkTopology.external  Rth=[.03, .2] K/W  Rth_Cauer=[.03, .1, .2] K/W  Rth_Foster=[.03, .2] K/W  thermal_mass_parameterization=ee.enum.thermalNetwork.thermalmass  thermal_mass=[3, 25] J/K  thermal_mass_Cauer=[3, 10, 25] J/K  thermal_mass_Foster=[33, 50] J/K  thermal_time_constant=[.1, 5] s  thermal_time_constant_Cauer=[.1, 1, 5] s  thermal_time_constant_Foster=[1, 10] s  thermal_mass_initial_temperatures=[80, 80] degC  thermal_mass_initial_temperatures_Cauer=[25, 25, 25] degC  junction_thermal_mass=JunctionTermalMass_m J/K  Tvec_initial_Foster=[25, 25, 25, 25] degC  RthDiode=[.03, .2] K/W  RthCauerDiode=[.03, .1, .2] K/W  RthFosterDiode=[.03, .2] K/W  thermalMassDiode=[3, 25] J/K  thermalMassCauerDiode=[3, 10, 25] J/K  thermalMassFosterDiode=[33, 50] J/K  thermalTauDiode=[.1, 5] s  thermalTauCauerDiode=[.1, 1, 5] s  thermalTauFosterDiode=[1, 10] s  thermalMassInitTempDiode=[25, 25] degC  thermalMassInitTempCauerDiode=[25, 25, 25] degC  junctionthermalMassDiode=0.1 J/K  TVecInitialFosterDiode=[25, 25, 25, 25] degC  no_thermal_network=0  mosfet_junction_temperature_specify=on  mosfet_junction_temperature_priority=High  mosfet_junction_temperature=Tambient_m+DThs_init_m degC  mosfet_junction_temperature_nominal_specify=off  mosfet_junction_temperature_nominal_value=1  mosfet_junction_temperature_nominal_unit=degC  diode_junction_temperature_specify=off  diode_junction_temperature_priority=None  diode_junction_temperature=25 degC  diode_junction_temperature_nominal_specify=off  diode_junction_temperature_nominal_value=1  diode_junction_temperature_nominal_unit=degC  Qj_specify=off  Qj_priority=None  Qj=0 W  Qj_nominal_specify=off  Qj_nominal_value=1  Qj_nominal_unit=W  accumulatedSwitchingLosses_specify=off  accumulatedSwitchingLosses_priority=None  accumulatedSwitchingLosses=0 J
  PS-Simulink Converter : nesl_utility/PS-Simulink Converter  PhysicalDomain=network_engine_domain  SubClassName=ps_output  LeftPortType=input  RightPortType=output  PseudoPeriodic=off  Frequencies=[]  VectorFormat=1-D array  Unit=W  AffineConversion=off
  PS-Simulink Converter1 : nesl_utility/PS-Simulink Converter  PhysicalDomain=network_engine_domain  SubClassName=ps_output  LeftPortType=input  RightPortType=output  PseudoPeriodic=off  Frequencies=[]  VectorFormat=1-D array  Unit=degC  AffineConversion=off
  PS-Simulink Converter2 : nesl_utility/PS-Simulink Converter  PhysicalDomain=network_engine_domain  SubClassName=ps_output  LeftPortType=input  RightPortType=output  PseudoPeriodic=off  Frequencies=[]  VectorFormat=1-D array  Unit=degC  AffineConversion=off
  Tambient : fl_lib/Thermal/Thermal Sources/Temperature Source  temperature=Tambient_m degC
  Temperature Sensor : fl_lib/Thermal/Thermal Sensors/Temperature Sensor  temperature_measure=foundation.enum.MeasurementReference.difference
  Temperature Sensor1 : fl_lib/Thermal/Thermal Sensors/Temperature Sensor  temperature_measure=foundation.enum.MeasurementReference.difference
  Voltage Sensor : fl_lib/Electrical/Electrical Sensors/Voltage Sensor
  heatsink_C : fl_lib/Thermal/Thermal Elements/Thermal Mass  mass_type=foundation.enum.constant_variable.constant  mass=mass_heatsink_m kg  sp_heat=specific_heat_m J/(K*kg)  mass_min=1e-6 kg  num_ports=foundation.enum.numPorts2.one  m_specify=off  m_priority=High  m=1 kg  m_nominal_specify=off  m_nominal_value=1  m_nominal_unit=kg  T_specify=on  T_priority=High  T=DThs_init_m+Tambient_m degC  T_nominal_specify=off  T_nominal_value=1  T_nominal_unit=K  Q_specify=off  Q_priority=High  Q=0 W  Q_nominal_specify=off  Q_nominal_value=1  Q_nominal_unit=W
  heatsink_R : fl_lib/Thermal/Thermal Elements/Thermal Resistance  resistance=rth_mosfet_HA_m K/W  T_specify=off  T_priority=High  T=0 deltadegC  T_nominal_specify=off  T_nominal_value=1  T_nominal_unit=K  Q_specify=off  Q_priority=None  Q=0 W  Q_nominal_specify=off  Q_nominal_value=1  Q_nominal_unit=W
  ic_zvs : nesl_utility/PS-Simulink Converter  PhysicalDomain=network_engine_domain  SubClassName=ps_output  LeftPortType=input  RightPortType=output  PseudoPeriodic=off  Frequencies=[]  VectorFormat=1-D array  Unit=A  AffineConversion=off
  iph1 : nesl_utility/PS-Simulink Converter  PhysicalDomain=network_engine_domain  SubClassName=ps_output  LeftPortType=input  RightPortType=output  PseudoPeriodic=off  Frequencies=[]  VectorFormat=1-D array  Unit=A  AffineConversion=off
  mosfet_sandwich : fl_lib/Thermal/Thermal Elements/Thermal Resistance  resistance=rth_mosfet_JH_m K/W  T_specify=off  T_priority=High  T=0 degC  T_nominal_specify=off  T_nominal_value=1  T_nominal_unit=K  Q_specify=off  Q_priority=None  Q=0 W  Q_nominal_specify=off  Q_nominal_value=1  Q_nominal_unit=W
  uph : nesl_utility/PS-Simulink Converter  PhysicalDomain=network_engine_domain  SubClassName=ps_output  LeftPortType=input  RightPortType=output  PseudoPeriodic=off  Frequencies=[]  VectorFormat=1-D array  Unit=V  AffineConversion=off
  G : PMIOPort  Side=Left
  D : PMIOPort  Port=2  Side=Left
  S : PMIOPort  Port=3  Side=Right
  tag scope: ic_zvs_Q2=scoped, mosfet_HA_temp_Q2=scoped, mosfet_JH_temp_Q2=scoped, mosfet_current_Q2=scoped, mosfet_ploss_Q2=scoped, mosfet_voltage_Q2=scoped
  wires:
  uph/1 -> [mosfet_voltage_Q2]  "uph"
  iph1/1 -> [mosfet_current_Q2]  "i_device_thermal_inv"
  PS-Simulink Converter1/1 -> [mosfet_JH_temp_Q2]  "mosfet_JH_temp"
  PS-Simulink Converter2/1 -> [mosfet_HA_temp_Q2]  "mosfet_HA_temp"
  PS-Simulink Converter/1 -> [mosfet_ploss_Q2]  "Power Losses"
  ic_zvs/1 -> [ic_zvs_Q2]  "ic_zvs"
  connections:
  Voltage Sensor/RConn1 -- uph/LConn1
  Current Sensor1/RConn1 -- iph1/LConn1
  Voltage Sensor/LConn1 -- Current Sensor2/LConn1 -- MOSFET/RConn1 -- Current Sensor1/RConn2
  Current Sensor1/LConn1 -- D/RConn1
  MOSFET/LConn2 -- Heat Flow Rate Sensor/LConn1
  Temperature Sensor1/RConn2 -- PS-Simulink Converter2/LConn1
  Temperature Sensor1/RConn1 -- heatsink_R/RConn1 -- Tambient/LConn1
  Temperature Sensor/RConn2 -- PS-Simulink Converter1/LConn1
  Temperature Sensor/RConn1 -- Temperature Sensor1/LConn1 -- mosfet_sandwich/RConn1 -- heatsink_R/LConn1 -- heatsink_C/LConn1
  Heat Flow Rate Sensor/RConn2 -- mosfet_sandwich/LConn1 -- Temperature Sensor/LConn1
  PS-Simulink Converter/LConn1 -- Heat Flow Rate Sensor/RConn1
  MOSFET/LConn1 -- G/RConn1
  Voltage Sensor/RConn2 -- Czvs/RConn1 -- MOSFET/RConn2 -- S/RConn1
  Czvs/LConn1 -- Current Sensor2/RConn2
  Current Sensor2/RConn1 -- ic_zvs/LConn1

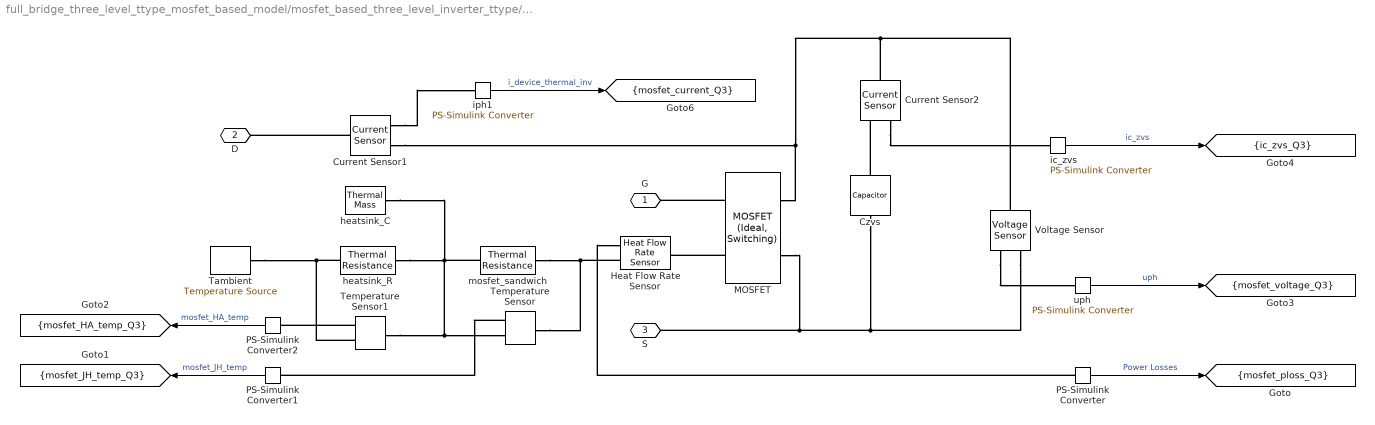
== system full_bridge_three_level_ttype_mosfet_based_model/mosfet_based_three_level_inverter_ttype/mosfet_thermal_3 ==
  Current Sensor1 : fl_lib/Electrical/Electrical Sensors/Current Sensor
  Current Sensor2 : fl_lib/Electrical/Electrical Sensors/Current Sensor
  Czvs : fl_lib/Electrical/Electrical Elements/Capacitor  c=Csnubber_m F  r=Rsnubber_m Ohm  g=0 1/Ohm  i_specify=off  i_priority=None  i=0 A  i_nominal_specify=off  i_nominal_value=1  i_nominal_unit=A  v_specify=off  v_priority=None  v=0 V  v_nominal_specify=off  v_nominal_value=1  v_nominal_unit=V  vc_specify=off  vc_priority=High  vc=0 V  vc_nominal_specify=off  vc_nominal_value=1  vc_nominal_unit=V
  Heat Flow Rate Sensor : fl_lib/Thermal/Thermal Sensors/Heat Flow Rate Sensor
  MOSFET : ee_lib/Semiconductors & Converters/MOSFET (Ideal, Switching)  port_option=ee.enum.controlport.ps  Rds=Rds_on_m Ohm  Goff=1e-6 1/Ohm  Vth=Vth_m V  diode_param=ee.enum.converters.protectiondiode.nodynamics  diode_Vf=Vdon_diode_m V  diode_Ron=Rdon_diode_m Ohm  diode_Goff=1e-5 1/Ohm  diode_C=50e-9 F  diode_iRM=-235 A  diode_iF=300 A  diode_idot=-50 A/us  diode_trr_param=ee.enum.converters.diodeReverseParam.trr_factor  diode_trr_factor=3  diode_trr=15 us  diode_Qrr=1500 s*uA  ids_specify=off  ids_priority=None  ids=0 A  ids_nominal_specify=off  ids_nominal_value=1  ids_nominal_unit=A  vds_specify=off  vds_priority=None  vds=0 V  vds_nominal_specify=off  vds_nominal_value=1  vds_nominal_unit=V  vgs_specify=off  vgs_priority=None  vgs=0 V  vgs_nominal_specify=off  vgs_nominal_value=1  vgs_nominal_unit=V  thermal_loss_option=ee.enum.converters.thermalLossOption.constantvalues  Von_data=[0, 1.8, 3.2, 6, 10, 16; 0, 2, 5.5, 9.5, 15, 25] V  Tj=[298.15, 448.15] K  Iout_data=[0, 20, 40, 60, 80, 100] A  tabulateWithVds=false  Eon_data=[0, 55.04, 124.57, 235.53, 362.12; 0, 71.25, 161.25, 304.88, 468.75] * 1e-6 J  Eoff_data=[0, 18, 30, 56.1, 76.5; 0, 22.5, 37.5, 70.13, 95.63] * 1e-6 J  Eon_data_3D=[zeros(2, 5, 3)] J  Eoff_data_3D=[zeros(2, 5, 3)] J  Tj_loss=[298.15, 448.15] K  Iout_data_loss=[0, 10, 20, 30, 40] A  Vds_loss=[0, 150, 300] V  Eon_scalar=Eon_m J  Eoff_scalar=Eoff_m J  Voff=Voff_sw_loss_m V  Iout_scalar=Ion_sw_loss_m A  useCurrentFromPreviousCycle=true  useVoltageFromPreviousCycle=true  diodeModelType=ee.enum.converters.diodeModelType.pwl  diodeTableType=ee.enum.diode.tableType.IfMat  diode_ReverseIVType=ee.enum.diode.diodeReverseIV.constant  diode_IfMat=[.07, .12, .19, 1.75, 4.24, 7.32, 11.2; .16, .3, .72, 2.14, 4.02, 6.35, 9.12] A  diode_VfMat=[.9, 1.15, 1.25, 1.5, 1.75, 2.17, 2.6, 2.85; .58, .68, .75, 1.1, 1.38, 1.77, 2.27, 2.7] V  diode_TjVec=[25, 125] degC  diode_VfVec=[.5, .7, .9, 1.3, 1.7, 2.1, 2.5] V  diode_IfVec=[.1, .2, .5, 1, 2, 4, 7, 10] A  diode_IrMat=[1e-06, 2e-06, 5e-06, 1e-05, 2.5e-05, 5e-05, .0001; 2e-06, 5e-06, 1e-05, 4e-05, 8e-05, .0002, .0005] A  diode_VrMat=[10, 100, 200, 250, 300, 325, 350; 10, 70, 160, 220, 270, 300, 320] V  diode_VrVec=[10, 20, 40, 50, 70, 80, 100] V  diode_IrVec=[1e-06, 2e-06, 5e-06, 1e-05, 2e-05, 5e-05, .0001] A  diode_Vr=-600 V  diode_Ls=150 nH  diode_Erec=0.03 J  diode_rec_loss_model=ee.enum.diode.reverseRecoveryModel.fixed  diode_ErecVal=0 J  diode_scaleWithIandV=false  diode_ErecMat=zeros(2, 3) J  diodeErecMat3D=zeros(2, 3, 2) J  diode_TjrecVec=[298.15, 398.15] K  diode_IfrecVec=[.1, 1, 10] A  diodeVrecVec=[0, 100] V  diode_IrecVal=10 A  diode_VrecVal=10 V  diode_tFilter=1 / 1000 / 100 s  separateThermalPortForDiode=false  thermal_network_parameterization=ee.enum.thermalNetworkTopology.external  Rth=[.03, .2] K/W  Rth_Cauer=[.03, .1, .2] K/W  Rth_Foster=[.03, .2] K/W  thermal_mass_parameterization=ee.enum.thermalNetwork.thermalmass  thermal_mass=[3, 25] J/K  thermal_mass_Cauer=[3, 10, 25] J/K  thermal_mass_Foster=[33, 50] J/K  thermal_time_constant=[.1, 5] s  thermal_time_constant_Cauer=[.1, 1, 5] s  thermal_time_constant_Foster=[1, 10] s  thermal_mass_initial_temperatures=[80, 80] degC  thermal_mass_initial_temperatures_Cauer=[25, 25, 25] degC  junction_thermal_mass=JunctionTermalMass_m J/K  Tvec_initial_Foster=[25, 25, 25, 25] degC  RthDiode=[.03, .2] K/W  RthCauerDiode=[.03, .1, .2] K/W  RthFosterDiode=[.03, .2] K/W  thermalMassDiode=[3, 25] J/K  thermalMassCauerDiode=[3, 10, 25] J/K  thermalMassFosterDiode=[33, 50] J/K  thermalTauDiode=[.1, 5] s  thermalTauCauerDiode=[.1, 1, 5] s  thermalTauFosterDiode=[1, 10] s  thermalMassInitTempDiode=[25, 25] degC  thermalMassInitTempCauerDiode=[25, 25, 25] degC  junctionthermalMassDiode=0.1 J/K  TVecInitialFosterDiode=[25, 25, 25, 25] degC  no_thermal_network=0  mosfet_junction_temperature_specify=on  mosfet_junction_temperature_priority=High  mosfet_junction_temperature=Tambient_m+DThs_init_m degC  mosfet_junction_temperature_nominal_specify=off  mosfet_junction_temperature_nominal_value=1  mosfet_junction_temperature_nominal_unit=degC  diode_junction_temperature_specify=off  diode_junction_temperature_priority=None  diode_junction_temperature=25 degC  diode_junction_temperature_nominal_specify=off  diode_junction_temperature_nominal_value=1  diode_junction_temperature_nominal_unit=degC  Qj_specify=off  Qj_priority=None  Qj=0 W  Qj_nominal_specify=off  Qj_nominal_value=1  Qj_nominal_unit=W  accumulatedSwitchingLosses_specify=off  accumulatedSwitchingLosses_priority=None  accumulatedSwitchingLosses=0 J
  PS-Simulink Converter : nesl_utility/PS-Simulink Converter  PhysicalDomain=network_engine_domain  SubClassName=ps_output  LeftPortType=input  RightPortType=output  PseudoPeriodic=off  Frequencies=[]  VectorFormat=1-D array  Unit=W  AffineConversion=off
  PS-Simulink Converter1 : nesl_utility/PS-Simulink Converter  PhysicalDomain=network_engine_domain  SubClassName=ps_output  LeftPortType=input  RightPortType=output  PseudoPeriodic=off  Frequencies=[]  VectorFormat=1-D array  Unit=degC  AffineConversion=off
  PS-Simulink Converter2 : nesl_utility/PS-Simulink Converter  PhysicalDomain=network_engine_domain  SubClassName=ps_output  LeftPortType=input  RightPortType=output  PseudoPeriodic=off  Frequencies=[]  VectorFormat=1-D array  Unit=degC  AffineConversion=off
  Tambient : fl_lib/Thermal/Thermal Sources/Temperature Source  temperature=Tambient_m degC
  Temperature Sensor : fl_lib/Thermal/Thermal Sensors/Temperature Sensor  temperature_measure=foundation.enum.MeasurementReference.difference
  Temperature Sensor1 : fl_lib/Thermal/Thermal Sensors/Temperature Sensor  temperature_measure=foundation.enum.MeasurementReference.difference
  Voltage Sensor : fl_lib/Electrical/Electrical Sensors/Voltage Sensor
  heatsink_C : fl_lib/Thermal/Thermal Elements/Thermal Mass  mass_type=foundation.enum.constant_variable.constant  mass=mass_heatsink_m kg  sp_heat=specific_heat_m J/(K*kg)  mass_min=1e-6 kg  num_ports=foundation.enum.numPorts2.one  m_specify=off  m_priority=High  m=1 kg  m_nominal_specify=off  m_nominal_value=1  m_nominal_unit=kg  T_specify=on  T_priority=High  T=DThs_init_m+Tambient_m degC  T_nominal_specify=off  T_nominal_value=1  T_nominal_unit=K  Q_specify=off  Q_priority=High  Q=0 W  Q_nominal_specify=off  Q_nominal_value=1  Q_nominal_unit=W
  heatsink_R : fl_lib/Thermal/Thermal Elements/Thermal Resistance  resistance=rth_mosfet_HA_m K/W  T_specify=off  T_priority=High  T=0 deltadegC  T_nominal_specify=off  T_nominal_value=1  T_nominal_unit=K  Q_specify=off  Q_priority=None  Q=0 W  Q_nominal_specify=off  Q_nominal_value=1  Q_nominal_unit=W
  ic_zvs : nesl_utility/PS-Simulink Converter  PhysicalDomain=network_engine_domain  SubClassName=ps_output  LeftPortType=input  RightPortType=output  PseudoPeriodic=off  Frequencies=[]  VectorFormat=1-D array  Unit=A  AffineConversion=off
  iph1 : nesl_utility/PS-Simulink Converter  PhysicalDomain=network_engine_domain  SubClassName=ps_output  LeftPortType=input  RightPortType=output  PseudoPeriodic=off  Frequencies=[]  VectorFormat=1-D array  Unit=A  AffineConversion=off
  mosfet_sandwich : fl_lib/Thermal/Thermal Elements/Thermal Resistance  resistance=rth_mosfet_JH_m K/W  T_specify=off  T_priority=High  T=0 degC  T_nominal_specify=off  T_nominal_value=1  T_nominal_unit=K  Q_specify=off  Q_priority=None  Q=0 W  Q_nominal_specify=off  Q_nominal_value=1  Q_nominal_unit=W
  uph : nesl_utility/PS-Simulink Converter  PhysicalDomain=network_engine_domain  SubClassName=ps_output  LeftPortType=input  RightPortType=output  PseudoPeriodic=off  Frequencies=[]  VectorFormat=1-D array  Unit=V  AffineConversion=off
  G : PMIOPort  Side=Left
  D : PMIOPort  Port=2  Side=Left
  S : PMIOPort  Port=3  Side=Right
  tag scope: ic_zvs_Q3=scoped, mosfet_HA_temp_Q3=scoped, mosfet_JH_temp_Q3=scoped, mosfet_current_Q3=scoped, mosfet_ploss_Q3=scoped, mosfet_voltage_Q3=scoped
  wires:
  PS-Simulink Converter/1 -> [mosfet_ploss_Q3]  "Power Losses"
  PS-Simulink Converter2/1 -> [mosfet_HA_temp_Q3]  "mosfet_HA_temp"
  PS-Simulink Converter1/1 -> [mosfet_JH_temp_Q3]  "mosfet_JH_temp"
  iph1/1 -> [mosfet_current_Q3]  "i_device_thermal_inv"
  uph/1 -> [mosfet_voltage_Q3]  "uph"
  ic_zvs/1 -> [ic_zvs_Q3]  "ic_zvs"
  connections:
  S/RConn1 -- MOSFET/RConn2 -- Czvs/RConn1 -- Voltage Sensor/RConn2
  MOSFET/LConn1 -- G/RConn1
  PS-Simulink Converter/LConn1 -- Heat Flow Rate Sensor/RConn1
  Temperature Sensor/LConn1 -- mosfet_sandwich/LConn1 -- Heat Flow Rate Sensor/RConn2
  Temperature Sensor1/LConn1 -- Temperature Sensor/RConn1 -- mosfet_sandwich/RConn1 -- heatsink_R/LConn1 -- heatsink_C/LConn1
  Temperature Sensor/RConn2 -- PS-Simulink Converter1/LConn1
  Temperature Sensor1/RConn1 -- heatsink_R/RConn1 -- Tambient/LConn1
  Temperature Sensor1/RConn2 -- PS-Simulink Converter2/LConn1
  MOSFET/LConn2 -- Heat Flow Rate Sensor/LConn1
  Current Sensor1/LConn1 -- D/RConn1
  Current Sensor1/RConn2 -- MOSFET/RConn1 -- Current Sensor2/LConn1 -- Voltage Sensor/LConn1
  Current Sensor1/RConn1 -- iph1/LConn1
  Voltage Sensor/RConn1 -- uph/LConn1
  Czvs/LConn1 -- Current Sensor2/RConn2
  Current Sensor2/RConn1 -- ic_zvs/LConn1
